simulink model "areaChange_"  (R2015a)
settings: Solver=FixedStepDiscrete  StartTime=0.0  StopTime=1.0  FixedStep=1.0  RelTol=1e-3
libraries: taXlibrary x8
settings Model: Creator=emmert  LastModifiedBy=thomas
settings DataIOCC: SignalLoggingSaveFormat=ModelDataLogs
settings OptimizationCC: ExpressionDepthLimit=2147483647
settings DebuggingCC: UnderspecifiedInitializationDetection=Classic  MergeDetectMultiDrivingBlocksExec=none  SolverPrmCheckMsg=warning  FcnCallInpInsideContextMsg=EnableAllAsWarning  StateNameClashWarn=warning
settings GRTTargetCC: CombineOutputUpdateFcns=off  GRTInterface=on

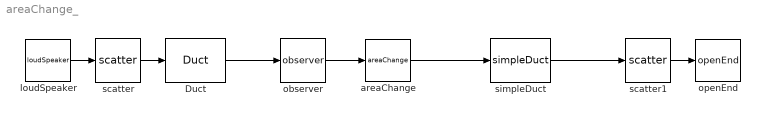
== system areaChange_ ==
  Duct : taXlibrary/Duct  element=Duct  order=3  minres=40  l=0.5  sensorPositions=[]
      settings: AttributesFormatString=%<l> m
  areaChange : taXlibrary/areaChange  element=lZeta  zeta=0  lred=0  leff=0  l=1  A=4
      settings: AttributesFormatString=%<A> m^2
  loudSpeaker : taXlibrary/loudSpeaker  element=loudSpeaker  loc=Upstream  Amp=1  A=1.4  Mach=0.1  rho=1.2  c=100
      settings: AttributesFormatString=%<Amp> m/s
  observer : taXlibrary/observer  element=observer  property=p_u
  openEnd : taXlibrary/openEnd  element=openEnd  loc=Downstream  A=[]  Mach=[]  rho=[]  c=[]
  scatter : taXlibrary/scatter  element=scatteringDummy  loc=Upstream
  scatter1 : taXlibrary/scatter  element=scatteringDummy  loc=Downstream
  simpleDuct : taXlibrary/simpleDuct  element=simpleDuct  l=0.25  damping_model_popup=no damping  gm=1.4  nu=1.568e-5  Pr=5  damping_model_id=1
      settings: AttributesFormatString=%<l> m
  wires:
  loudSpeaker/1 -> scatter/1
  scatter/1 -> Duct/1
  scatter1/1 -> openEnd/1
  observer/1 -> areaChange/1
  Duct/1 -> observer/1
  areaChange/1 -> simpleDuct/1
  simpleDuct/1 -> scatter1/1
